simulink model "SF045A_HwAgSysArbn"  (R2013b)
settings: Solver=FixedStepDiscrete  SolverMode=SingleTasking  StartTime=0.0  StopTime=1  FixedStep=.002  RelTol=1e-3
values from neighbouring files (symbols this model uses):
  ARCHGLBPRM_2MILLISEC_SEC_F32 = DataDict.Constant    [SF045A_HwAgSysArbn_DataDict.m]
  CNVSECTOCNT_CNTPERSEC_U32 = DataDict.Constant    [SF045A_HwAgSysArbn_DataDict.m]
  CNVTOMILLISEC_MILLISECPERCNT_F32 = DataDict.Constant    [SF045A_HwAgSysArbn_DataDict.m]
  FltInj_f32 = DataDict.Client    [SF045A_HwAgSysArbn_DataDict.m]
  FLTINJ_HWAGSYSARBN_HWAG = DataDict.Constant    [SF045A_HwAgSysArbn_DataDict.m]
  FLTINJ_HWAGSYSARBN_SERLCOMHWAG = DataDict.Constant    [SF045A_HwAgSysArbn_DataDict.m]
  HwAgSysArbnHwAgConf1Snsr = DataDict.Calibration    [SF045A_HwAgSysArbn_DataDict.m]
  HwAgSysArbnHwAgConf2Snsr = DataDict.Calibration    [SF045A_HwAgSysArbn_DataDict.m]
  HwAgSysArbnHwAgConfNoSnsr = DataDict.Calibration    [SF045A_HwAgSysArbn_DataDict.m]
  HwAgSysArbnHwAgCorrdCorrlnThd = DataDict.Calibration    [SF045A_HwAgSysArbn_DataDict.m]
  HwAgSysArbnHwAgCorrlnFailDebStep = DataDict.Calibration    [SF045A_HwAgSysArbn_DataDict.m]
  HwAgSysArbnHwAgCorrlnPassDebStep = DataDict.Calibration    [SF045A_HwAgSysArbn_DataDict.m]
  HwAgSysArbnHwAgCorrlnRng = DataDict.Calibration    [SF045A_HwAgSysArbn_DataDict.m]
  HwAgSysArbnHwAgSlewRate = DataDict.Calibration    [SF045A_HwAgSysArbn_DataDict.m]
  HwAgSysArbnHwAgSnsrlsCorrlnThd = DataDict.Calibration    [SF045A_HwAgSysArbn_DataDict.m]
  HwAgSysArbnHwAgSnsrlsKineThd = DataDict.Calibration    [SF045A_HwAgSysArbn_DataDict.m]
  HwAgSysArbnHwAgToMotAgCorrlnElpdTiLim = DataDict.Calibration    [SF045A_HwAgSysArbn_DataDict.m]
  HwAgSysArbnSerlComHwAgCorrdConf = DataDict.Calibration    [SF045A_HwAgSysArbn_DataDict.m]
  HwAgSysArbnSerlComHwAgSnsrlsConf = DataDict.Calibration    [SF045A_HwAgSysArbn_DataDict.m]
  HwAgSysArbnSlewRateTmr = DataDict.Calibration    [SF045A_HwAgSysArbn_DataDict.m]
  HWAGTHD_ULS_FLOAT32 = DataDict.Constant    [SF045A_HwAgSysArbn_DataDict.m]
  INVLDSRC_CNT_S08 = DataDict.Constant    [SF045A_HwAgSysArbn_DataDict.m]
  LRGSLEW_HWDEGPERSEC_F32 = DataDict.Constant    [SF045A_HwAgSysArbn_DataDict.m]
  NODEBSTEP_CNT_U16 = DataDict.Constant    [SF045A_HwAgSysArbn_DataDict.m]
  SLEWINPROGS_CNT_LGC = DataDict.Constant    [SF045A_HwAgSysArbn_DataDict.m]
  SLEWNOTINPROGS_CNT_LGC = DataDict.Constant    [SF045A_HwAgSysArbn_DataDict.m]
  SNSRDATASRCSELD_CNT_S08 = DataDict.Constant    [SF045A_HwAgSysArbn_DataDict.m]
  SNSRLSDATASRCSELD_CNT_S08 = DataDict.Constant    [SF045A_HwAgSysArbn_DataDict.m]
  ZEROTMR_MILLISEC_F32 = DataDict.Constant    [SF045A_HwAgSysArbn_DataDict.m]
undefined symbols (not defined in the file or in its folder): NtcNr1, NtcSts1
libraries: simulink x10, NxtrLim x7, autosarlib x2, NxtrAbslt x2
(part 3 of 3)

== system SF045A_HwAgSysArbn/HwAgSysArbn/HwAgSysArbnPer1/HwAgArbn/HwAgSrcSeln/ChkCorrln/SetNtcPass ==
  Action Port : ActionPort  ActionType=then
  Constant15 : Constant  RequirementInfo={} %GIDa_eeb50086_ebb6_4513_9847_6cae94a7ac91  Value=HwAgSysArbnHwAgCorrlnPassDebStep
  Constant18 : Constant  RequirementInfo={} %GIDa_013e9517_c477_4830_bdf4_1b47d908796e  Value=0
  Constant4 : Constant  RequirementInfo={} %GIDa_90515fd1_2125_4550_9fa1_625f6dc30aa8  Value=true  OutDataTypeStr=boolean
      settings: AttributesFormatString=%<OutDataTypeStr>
  CopyRight2 : Subsystem  Description=|  mask(Copyright Information){none=on}
      | Copyright info block.                                               
      |                                                                     
      | Place copyright information at the top of every subsystem in design.
      mask prompts: none "No parameters"
      mask help: Place copyright information at the top of every subsystem in design.
      mask Display:
      | NxtrConf = 'Nexteer Confidential';
      | 
      | sys = bdroot; %handle for the current model ("system")
      | first = get_param(sys,'Created');
      | first = first(end-3:end);  %year is last four digits
      | 
      | last = get_param(sys,'LastModifiedDate');
      | if isempty(last)
      |     last = datestr(now,'yyyy');
      | else
      |     last = last(end-3:end);
      | end
      | 
      | if strcmp(first,last)
      |     fprintf('%s -- Copyright %s Nexteer',NxtrConf,first)
      | else
      |     fprintf('%s -- %s%s- %s Nexteer',NxtrConf,char(169),first,last)
      | end
  Data Store Write1 : DataStoreWrite  RequirementInfo={} %GIDa_5a1ff29e_b92d_44ac_baea_bdad4ffa5dd1  DataStoreName=HwAgToMotAgCorrlnDurnRefTmr
  Data Store Write3 : DataStoreWrite  RequirementInfo={} %GIDa_9a2b2c1d_b743_4844_a03a_8556aaa946e3  DataStoreName=HwAgToMotAgCorrln
  Enumerated Constant13 : simulink/Sources/Enumerated Constant  RequirementInfo={} %GIDa_0b00377d_3f79_4e44_b7d4_456cdb84d0e3  OutDataTypeStr=Enum: NtcSts1  Value=NtcSts1.NTCSTS_PREPASSD  SampleTime=inf
  Enumerated Constant15 : simulink/Sources/Enumerated Constant  RequirementInfo={} %GIDa_b1678220_307d_46cf_99b1_3b05cdcccb07  OutDataTypeStr=Enum: NtcNr1  Value=NtcNr1.NTCNR_0X0A6  SampleTime=inf
  GetRefTmr100MicroSec32bit : Subsystem  RequirementInfo={} %GIDa_050abb2d_d94a_4647_9003_ba1ceee815fb
  SetNtcPass : Subsystem  RequirementInfo={} %GIDa_56eadc5f_fb1c_4ab9_8fbe_9c5bb2cbb9bf  mask(SetNTC){}
      mask help: SetNTC library block
  wires:
  Constant15/1 -> SetNtcPass/4(DebStep)
  Enumerated Constant13/1 -> SetNtcPass/3(NtcSts)
  Constant18/1 -> SetNtcPass/2(NtcStInfo)
  Enumerated Constant15/1 -> SetNtcPass/1(NtcNr)
  Constant4/1 -> Data Store Write3/1
  GetRefTmr100MicroSec32bit/1(RefTmr) -> Data Store Write1/1

== system SF045A_HwAgSysArbn/HwAgSysArbn/HwAgSysArbnPer1/HwAgArbn/HwAgSrcSeln/NoHwAgDataToSerlCom/CopyRight2 ==

== system SF045A_HwAgSysArbn/HwAgSysArbn/HwAgSysArbnPer1/HwAgArbn/HwAgSrcSeln/SnsrDataToSerlCom/CopyRight2 ==

== system SF045A_HwAgSysArbn/HwAgSysArbn/HwAgSysArbnPer1/HwAgArbn/HwAgSrcSeln/SnsrlsDataToSerlCom/CopyRight2 ==

== system SF045A_HwAgSysArbn/HwAgSysArbn/HwAgSysArbnPer1/HwAgArbn/HwAgSrcSeln/SnsrlsDataToSerlCom/CorrlnStsFalse ==
  Action Port : ActionPort  ActionType=else
  Constant1 : Constant  RequirementInfo={} %GIDa_c7135156_251f_40b0_8356_b5a0132d025b  Value=0  OutDataTypeStr=single
      settings: AttributesFormatString=%<OutDataTypeStr>
  Constant3 : Constant  RequirementInfo={} %GIDa_afd38917_26d9_466b_8fc0_bc806b5335e9  Value=0  OutDataTypeStr=boolean
      settings: AttributesFormatString=%<OutDataTypeStr>
  CopyRight2 : Subsystem  Description=|  mask(Copyright Information){none=on}
      | Copyright info block.                                               
      |                                                                     
      | Place copyright information at the top of every subsystem in design.
      mask prompts: none "No parameters"
      mask help: Place copyright information at the top of every subsystem in design.
      mask Display:
      | NxtrConf = 'Nexteer Confidential';
      | 
      | sys = bdroot; %handle for the current model ("system")
      | first = get_param(sys,'Created');
      | first = first(end-3:end);  %year is last four digits
      | 
      | last = get_param(sys,'LastModifiedDate');
      | if isempty(last)
      |     last = datestr(now,'yyyy');
      | else
      |     last = last(end-3:end);
      | end
      | 
      | if strcmp(first,last)
      |     fprintf('%s -- Copyright %s Nexteer',NxtrConf,first)
      | else
      |     fprintf('%s -- %s%s- %s Nexteer',NxtrConf,char(169),first,last)
      | end
  HwAgToSerlCom : Outport  RequirementInfo={} %GIDa_dfac9b99_a6ce_41fa_a1af_5a78eaec718f
  HwAgStsToSerlCom : Outport  RequirementInfo={} %GIDa_a5794653_43a3_4f48_8d32_c475f5222fa0  Port=2
  wires:
  Constant3/1 -> HwAgStsToSerlCom/1
  Constant1/1 -> HwAgToSerlCom/1

== system SF045A_HwAgSysArbn/HwAgSysArbn/HwAgSysArbnPer1/HwAgArbn/HwAgSrcSeln/SnsrlsDataToSerlCom/CorrlnStsTrue ==
  HwAgSnsrls : Inport
  HwAgSnsrlsConf : Inport  Port=2
  Action Port : ActionPort  ActionType=then
  Constant8 : Constant  RequirementInfo={} %GIDa_349ca605_e3c4_4ce4_8a04_8b4b7b6ac69d  Value=HwAgSysArbnSerlComHwAgSnsrlsConf
  CopyRight2 : Subsystem  Description=|  mask(Copyright Information){none=on}
      | Copyright info block.                                               
      |                                                                     
      | Place copyright information at the top of every subsystem in design.
      mask prompts: none "No parameters"
      mask help: Place copyright information at the top of every subsystem in design.
      mask Display:
      | NxtrConf = 'Nexteer Confidential';
      | 
      | sys = bdroot; %handle for the current model ("system")
      | first = get_param(sys,'Created');
      | first = first(end-3:end);  %year is last four digits
      | 
      | last = get_param(sys,'LastModifiedDate');
      | if isempty(last)
      |     last = datestr(now,'yyyy');
      | else
      |     last = last(end-3:end);
      | end
      | 
      | if strcmp(first,last)
      |     fprintf('%s -- Copyright %s Nexteer',NxtrConf,first)
      | else
      |     fprintf('%s -- %s%s- %s Nexteer',NxtrConf,char(169),first,last)
      | end
  Relational Operator : RelationalOperator  RequirementInfo={} %GIDa_03f84a5a_5c25_4fbe_b033_45a585c8ca69  OutDataTypeStr=boolean
  HwAgToSerlCom : Outport
  HwAgStsToSerlCom : Outport  Port=2
  wires:
  Relational Operator/1 -> HwAgStsToSerlCom/1
  Constant8/1 -> Relational Operator/2
  HwAgSnsrlsConf/1 -> Relational Operator/1
  HwAgSnsrls/1 -> HwAgToSerlCom/1

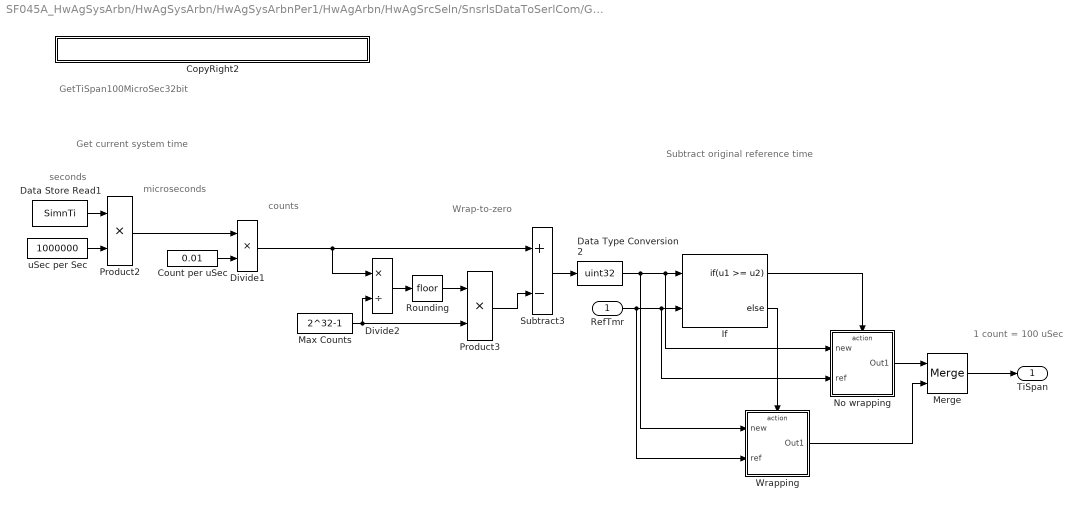
== system SF045A_HwAgSysArbn/HwAgSysArbn/HwAgSysArbnPer1/HwAgArbn/HwAgSrcSeln/SnsrlsDataToSerlCom/GetTiSpan100MicroSec32bit ==
  note: Subtract original reference time
  note: seconds
  note: microseconds
  note: counts
  note: Wrap-to-zero
  note: 1 count = 100 uSec
  note: Get current system time
  note: GetTiSpan100MicroSec32bit
  RefTmr : Inport
  CopyRight2 : Subsystem  Description=|  mask(Copyright Information){none=on}
      | Copyright info block.                                               
      |                                                                     
      | Place copyright information at the top of every subsystem in design.
      mask prompts: none "No parameters"
      mask help: Place copyright information at the top of every subsystem in design.
      mask Display:
      | NxtrConf = 'Nexteer Confidential';
      | 
      | sys = bdroot; %handle for the current model ("system")
      | first = get_param(sys,'Created');
      | if(isempty(first))
      |     first = datestr(now,'yyyy');
      | else
      |     first = first(end-3:end);  %year is last four digits
      | end
      | 
      | last = get_param(sys,'LastModifiedDate');
      | if isempty(last)
      |     last = datestr(now,'yyyy');
      | else
      |     last = last(end-3:end);
      | end
      | 
      | if strcmp(first,last)
      |     fprintf('%s -- Copyright %s Nexteer',NxtrConf,first)
      | else
      |     fprintf('%s -- %s%s- %s Nexteer',NxtrConf,char(169),first,last)
      | end
  Count per uSec : Constant  Value=0.01
  Data Store Read1 : DataStoreRead  DataStoreName=SimnTi
  Data Type Conversion2 : DataTypeConversion  OutDataTypeStr=uint32
  Divide1 : Product  Inputs=**
  Divide2 : Product  Inputs=*/
  If : If  NumInputs=2  IfExpression=u1 >= u2
  Max Counts : Constant  Value=2^32-1
  Merge : Merge
  No wrapping : Subsystem  TreatAsAtomicUnit=on
  Product2 : Product
  Product3 : Product
  Rounding : Rounding
  Subtract3 : Sum  Inputs=+-
  Wrapping : Subsystem  TreatAsAtomicUnit=on
  uSec per Sec : Constant  Value=1000000
  TiSpan : Outport
  wires:
  Wrapping/1(Out1) -> Merge/2
  No wrapping/1(Out1) -> Merge/1
  If/2 -> Wrapping/Action
  If/1 -> No wrapping/Action
  Product3/1 -> Subtract3/2
  Subtract3/1 -> Data Type Conversion2/1
  Rounding/1 -> Product3/1
  Divide2/1 -> Rounding/1
  Max Counts/1 -> Divide2/2, Product3/2
  Divide1/1 -> Divide2/1, Subtract3/1
  Product2/1 -> Divide1/1
  Data Store Read1/1 -> Product2/1
  Count per uSec/1 -> Divide1/2
  uSec per Sec/1 -> Product2/2
  Merge/1 -> TiSpan/1
  RefTmr/1 -> If/2, No wrapping/2(ref), Wrapping/2(ref)
  Data Type Conversion2/1 -> If/1, No wrapping/1(new), Wrapping/1(new)

== system SF045A_HwAgSysArbn/HwAgSysArbn/HwAgSysArbnPer1/HwAgArbn/HwAgSrcSeln/SnsrlsHwAgSeln/CopyRight2 ==

== system SF045A_HwAgSysArbn/HwAgSysArbn/HwAgSysArbnPer1/HwAgArbn/HwAgSrcSeln/VrfyHwAgCorrln/CopyRight2 ==

== system SF045A_HwAgSysArbn/HwAgSysArbn/HwAgSysArbnPer1/HwAgArbn/TestHwAgSrcChg/ RetainSlewRate/CopyRight2 ==

== system SF045A_HwAgSysArbn/HwAgSysArbn/HwAgSysArbnPer1/HwAgArbn/TestHwAgSrcChg/ApplyLrgSlew/CopyRight2 ==

== system SF045A_HwAgSysArbn/HwAgSysArbn/HwAgSysArbnPer1/HwAgArbn/TestHwAgSrcChg/ApplyRateLim/ RetainHwAgConf ==
  note: Pass on the previous values of Hw Ag Confidence as Slewing is not complete
  PrevHwAgConf : Inport
  Action Port : ActionPort  ActionType=then
  Constant4 : Constant  Value=SLEWINPROGS_CNT_LGC
  CopyRight2 : Subsystem  Description=|  mask(Copyright Information){none=on}
      | Copyright info block.                                               
      |                                                                     
      | Place copyright information at the top of every subsystem in design.
      mask prompts: none "No parameters"
      mask help: Place copyright information at the top of every subsystem in design.
      mask Display:
      | NxtrConf = 'Nexteer Confidential';
      | 
      | sys = bdroot; %handle for the current model ("system")
      | first = get_param(sys,'Created');
      | first = first(end-3:end);  %year is last four digits
      | 
      | last = get_param(sys,'LastModifiedDate');
      | if isempty(last)
      |     last = datestr(now,'yyyy');
      | else
      |     last = last(end-3:end);
      | end
      | 
      | if strcmp(first,last)
      |     fprintf('%s -- Copyright %s Nexteer',NxtrConf,first)
      | else
      |     fprintf('%s -- %s%s- %s Nexteer',NxtrConf,char(169),first,last)
      | end
  Data Store Write5 : DataStoreWrite  RequirementInfo={} %GIDa_e610268f_4251_4a50_930a_b136411808b8  DataStoreName=SlewSts
  "HwAgConf " : Outport
  wires:
  PrevHwAgConf/1 -> "HwAgConf "/1
  Constant4/1 -> Data Store Write5/1

== system SF045A_HwAgSysArbn/HwAgSysArbn/HwAgSysArbnPer1/HwAgArbn/TestHwAgSrcChg/ApplyRateLim/CopyRight2 ==

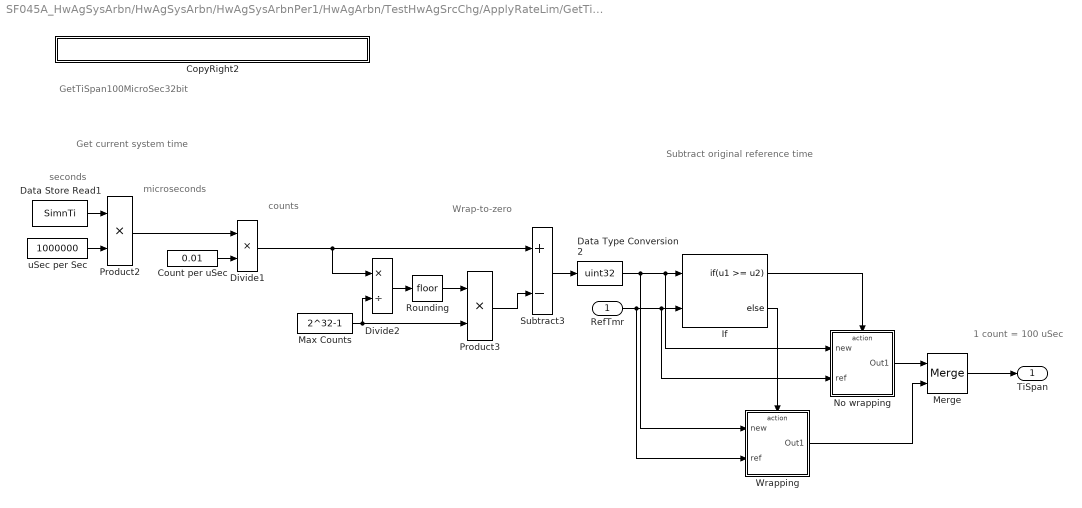
== system SF045A_HwAgSysArbn/HwAgSysArbn/HwAgSysArbnPer1/HwAgArbn/TestHwAgSrcChg/ApplyRateLim/GetTiSpan100MicroSec32bit ==
  note: Subtract original reference time
  note: seconds
  note: microseconds
  note: counts
  note: Wrap-to-zero
  note: 1 count = 100 uSec
  note: Get current system time
  note: GetTiSpan100MicroSec32bit
  RefTmr : Inport
  CopyRight2 : Subsystem  Description=|  mask(Copyright Information){none=on}
      | Copyright info block.                                               
      |                                                                     
      | Place copyright information at the top of every subsystem in design.
      mask prompts: none "No parameters"
      mask help: Place copyright information at the top of every subsystem in design.
      mask Display:
      | NxtrConf = 'Nexteer Confidential';
      | 
      | sys = bdroot; %handle for the current model ("system")
      | first = get_param(sys,'Created');
      | if(isempty(first))
      |     first = datestr(now,'yyyy');
      | else
      |     first = first(end-3:end);  %year is last four digits
      | end
      | 
      | last = get_param(sys,'LastModifiedDate');
      | if isempty(last)
      |     last = datestr(now,'yyyy');
      | else
      |     last = last(end-3:end);
      | end
      | 
      | if strcmp(first,last)
      |     fprintf('%s -- Copyright %s Nexteer',NxtrConf,first)
      | else
      |     fprintf('%s -- %s%s- %s Nexteer',NxtrConf,char(169),first,last)
      | end
  Count per uSec : Constant  Value=0.01
  Data Store Read1 : DataStoreRead  DataStoreName=SimnTi
  Data Type Conversion2 : DataTypeConversion  OutDataTypeStr=uint32
  Divide1 : Product  Inputs=**
  Divide2 : Product  Inputs=*/
  If : If  NumInputs=2  IfExpression=u1 >= u2
  Max Counts : Constant  Value=2^32-1
  Merge : Merge
  No wrapping : Subsystem  TreatAsAtomicUnit=on
  Product2 : Product
  Product3 : Product
  Rounding : Rounding
  Subtract3 : Sum  Inputs=+-
  Wrapping : Subsystem  TreatAsAtomicUnit=on
  uSec per Sec : Constant  Value=1000000
  TiSpan : Outport
  wires:
  Wrapping/1(Out1) -> Merge/2
  No wrapping/1(Out1) -> Merge/1
  If/2 -> Wrapping/Action
  If/1 -> No wrapping/Action
  Product3/1 -> Subtract3/2
  Subtract3/1 -> Data Type Conversion2/1
  Rounding/1 -> Product3/1
  Divide2/1 -> Rounding/1
  Max Counts/1 -> Divide2/2, Product3/2
  Divide1/1 -> Divide2/1, Subtract3/1
  Product2/1 -> Divide1/1
  Data Store Read1/1 -> Product2/1
  Count per uSec/1 -> Divide1/2
  uSec per Sec/1 -> Product2/2
  Merge/1 -> TiSpan/1
  RefTmr/1 -> If/2, No wrapping/2(ref), Wrapping/2(ref)
  Data Type Conversion2/1 -> If/1, No wrapping/1(new), Wrapping/1(new)

== system SF045A_HwAgSysArbn/HwAgSysArbn/HwAgSysArbnPer1/HwAgArbn/TestHwAgSrcChg/ApplyRateLim/Pass ==
  note: Pass on the computed values of Hw Ag Confidence as Slewing is not in progress
  HwAgConfInp : Inport
  Action Port : ActionPort  ActionType=else
  Constant4 : Constant  Value=SLEWNOTINPROGS_CNT_LGC
  CopyRight2 : Subsystem  Description=|  mask(Copyright Information){none=on}
      | Copyright info block.                                               
      |                                                                     
      | Place copyright information at the top of every subsystem in design.
      mask prompts: none "No parameters"
      mask help: Place copyright information at the top of every subsystem in design.
      mask Display:
      | NxtrConf = 'Nexteer Confidential';
      | 
      | sys = bdroot; %handle for the current model ("system")
      | first = get_param(sys,'Created');
      | first = first(end-3:end);  %year is last four digits
      | 
      | last = get_param(sys,'LastModifiedDate');
      | if isempty(last)
      |     last = datestr(now,'yyyy');
      | else
      |     last = last(end-3:end);
      | end
      | 
      | if strcmp(first,last)
      |     fprintf('%s -- Copyright %s Nexteer',NxtrConf,first)
      | else
      |     fprintf('%s -- %s%s- %s Nexteer',NxtrConf,char(169),first,last)
      | end
  Data Store Write5 : DataStoreWrite  RequirementInfo={} %GIDa_e00d6d32_3e14_4362_9726_dd90d4df3b91  DataStoreName=SlewSts
  "HwAgConf " : Outport
  wires:
  HwAgConfInp/1 -> "HwAgConf "/1
  Constant4/1 -> Data Store Write5/1

== system SF045A_HwAgSysArbn/HwAgSysArbn/HwAgSysArbnPer1/HwAgArbn/TestHwAgSrcChg/SetSlewRate/CopyRight2 ==

== system SF045A_HwAgSysArbn/HwAgSysArbn/HwAgSysArbnPer1/HwAgArbn/TestHwAgSrcChg/SetSlewRate/GetRefTmr100MicroSec32bit ==
  note: 1 count = 100 uSec
  note: seconds
  note: microseconds
  note: counts
  note: Wrap-to-zero
  note: GetRefTmr100MicroSec32bit
  CopyRight2 : Subsystem  Description=|  mask(Copyright Information){none=on}
      | Copyright info block.                                               
      |                                                                     
      | Place copyright information at the top of every subsystem in design.
      mask prompts: none "No parameters"
      mask help: Place copyright information at the top of every subsystem in design.
      mask Display:
      | NxtrConf = 'Nexteer Confidential';
      | 
      | sys = bdroot; %handle for the current model ("system")
      | first = get_param(sys,'Created');
      | if(isempty(first))
      |     first = datestr(now,'yyyy');
      | else
      |     first = first(end-3:end);  %year is last four digits
      | end
      | 
      | last = get_param(sys,'LastModifiedDate');
      | if isempty(last)
      |     last = datestr(now,'yyyy');
      | else
      |     last = last(end-3:end);
      | end
      | 
      | if strcmp(first,last)
      |     fprintf('%s -- Copyright %s Nexteer',NxtrConf,first)
      | else
      |     fprintf('%s -- %s%s- %s Nexteer',NxtrConf,char(169),first,last)
      | end
  Count per uSec : Constant  Value=0.01
  Data Store Read1 : DataStoreRead  DataStoreName=SimnTi
  Data Type Conversion1 : DataTypeConversion  OutDataTypeStr=uint32
  Divide1 : Product  Inputs=**
  Divide2 : Product  Inputs=*/
  Max Counts : Constant  Value=2^32-1
  Product1 : Product
  Product2 : Product
  Rounding : Rounding
  Subtract1 : Sum  Inputs=+-
  uSec per Sec : Constant  Value=1000000
  RefTmr : Outport
  wires:
  Product2/1 -> Subtract1/2
  Subtract1/1 -> Data Type Conversion1/1
  Rounding/1 -> Product2/1
  Divide2/1 -> Rounding/1
  Max Counts/1 -> Divide2/2, Product2/2
  Divide1/1 -> Divide2/1, Subtract1/1
  Product1/1 -> Divide1/1
  Data Store Read1/1 -> Product1/1
  Count per uSec/1 -> Divide1/2
  uSec per Sec/1 -> Product1/2
  Data Type Conversion1/1 -> RefTmr/1

== system SF045A_HwAgSysArbn/HwAgSysArbn/HwAgSysArbnPer1/HwAgArbn/VldtSnsrlsData/Pass/CopyRight2 ==

== system SF045A_HwAgSysArbn/HwAgSysArbn/HwAgSysArbnPer1/HwAgArbn/VldtSnsrlsData/ThdExcdd/CopyRight2 ==

== system SF045A_HwAgSysArbn/HwAgSysArbn/HwAgSysArbnPer1/HwAgArbn/VldtSnsrlsData/ThdExcdd/Kinematic Integrity ==
  NtcNr : Inport
  NtcStInfo : Inport  Port=2
  NtcSts : Inport  Port=3
  DebStep : Inport  Port=4
  SetNtcSts : Subsystem  RequirementInfo={} %GIDa_58144789_61c4_4a7b_8c14_60385a32cfb3  TreatAsAtomicUnit=on
      settings: RTWSystemCode=Inline
  wires:
  NtcStInfo/1 -> SetNtcSts/2(NtcStInfo)
  DebStep/1 -> SetNtcSts/4(DebStep)
  NtcSts/1 -> SetNtcSts/3(NtcSts)
  NtcNr/1 -> SetNtcSts/1(NtcNr)  "NtcNr"

== system SF045A_HwAgSysArbn/HwAgSysArbn/HwAgSysArbnPer1/HwAgArbn/HwAgSrcSeln/ChkCorrln/SetCorrlFltNtc/CopyRight2 ==

== system SF045A_HwAgSysArbn/HwAgSysArbn/HwAgSysArbnPer1/HwAgArbn/HwAgSrcSeln/ChkCorrln/SetCorrlFltNtc/SetCorrlFltNtc ==
  NtcNr : Inport
  NtcStInfo : Inport  Port=2
  NtcSts : Inport  Port=3
  DebStep : Inport  Port=4
  SetNtcSts : Subsystem  RequirementInfo={} %GIDa_0a5e138f_bbbe_4d9e_8ebe_c8090c91025c  TreatAsAtomicUnit=on
      settings: RTWSystemCode=Inline
  wires:
  NtcStInfo/1 -> SetNtcSts/2(NtcStInfo)
  DebStep/1 -> SetNtcSts/4(DebStep)
  NtcSts/1 -> SetNtcSts/3(NtcSts)
  NtcNr/1 -> SetNtcSts/1(NtcNr)  "NtcNr"

== system SF045A_HwAgSysArbn/HwAgSysArbn/HwAgSysArbnPer1/HwAgArbn/HwAgSrcSeln/ChkCorrln/SetNtcPass/CopyRight2 ==

== system SF045A_HwAgSysArbn/HwAgSysArbn/HwAgSysArbnPer1/HwAgArbn/HwAgSrcSeln/ChkCorrln/SetNtcPass/GetRefTmr100MicroSec32bit ==
  note: 1 count = 100 uSec
  note: seconds
  note: microseconds
  note: counts
  note: Wrap-to-zero
  note: GetRefTmr100MicroSec32bit
  CopyRight2 : Subsystem  Description=|  mask(Copyright Information){none=on}
      | Copyright info block.                                               
      |                                                                     
      | Place copyright information at the top of every subsystem in design.
      mask prompts: none "No parameters"
      mask help: Place copyright information at the top of every subsystem in design.
      mask Display:
      | NxtrConf = 'Nexteer Confidential';
      | 
      | sys = bdroot; %handle for the current model ("system")
      | first = get_param(sys,'Created');
      | if(isempty(first))
      |     first = datestr(now,'yyyy');
      | else
      |     first = first(end-3:end);  %year is last four digits
      | end
      | 
      | last = get_param(sys,'LastModifiedDate');
      | if isempty(last)
      |     last = datestr(now,'yyyy');
      | else
      |     last = last(end-3:end);
      | end
      | 
      | if strcmp(first,last)
      |     fprintf('%s -- Copyright %s Nexteer',NxtrConf,first)
      | else
      |     fprintf('%s -- %s%s- %s Nexteer',NxtrConf,char(169),first,last)
      | end
  Count per uSec : Constant  Value=0.01
  Data Store Read1 : DataStoreRead  DataStoreName=SimnTi
  Data Type Conversion1 : DataTypeConversion  OutDataTypeStr=uint32
  Divide1 : Product  Inputs=**
  Divide2 : Product  Inputs=*/
  Max Counts : Constant  Value=2^32-1
  Product1 : Product
  Product2 : Product
  Rounding : Rounding
  Subtract1 : Sum  Inputs=+-
  uSec per Sec : Constant  Value=1000000
  RefTmr : Outport
  wires:
  Product2/1 -> Subtract1/2
  Subtract1/1 -> Data Type Conversion1/1
  Rounding/1 -> Product2/1
  Divide2/1 -> Rounding/1
  Max Counts/1 -> Divide2/2, Product2/2
  Divide1/1 -> Divide2/1, Subtract1/1
  Product1/1 -> Divide1/1
  Data Store Read1/1 -> Product1/1
  Count per uSec/1 -> Divide1/2
  uSec per Sec/1 -> Product1/2
  Data Type Conversion1/1 -> RefTmr/1

== system SF045A_HwAgSysArbn/HwAgSysArbn/HwAgSysArbnPer1/HwAgArbn/HwAgSrcSeln/ChkCorrln/SetNtcPass/SetNtcPass ==
  NtcNr : Inport
  NtcStInfo : Inport  Port=2
  NtcSts : Inport  Port=3
  DebStep : Inport  Port=4
  SetNtcSts : Subsystem  RequirementInfo={} %GIDa_17711836_ebc0_49f1_9698_b758e03a4efd  TreatAsAtomicUnit=on
      settings: RTWSystemCode=Inline
  wires:
  NtcNr/1 -> SetNtcSts/1(NtcNr)  "NtcNr"
  NtcSts/1 -> SetNtcSts/3(NtcSts)
  DebStep/1 -> SetNtcSts/4(DebStep)
  NtcStInfo/1 -> SetNtcSts/2(NtcStInfo)

== system SF045A_HwAgSysArbn/HwAgSysArbn/HwAgSysArbnPer1/HwAgArbn/HwAgSrcSeln/SnsrlsDataToSerlCom/CorrlnStsFalse/CopyRight2 ==

== system SF045A_HwAgSysArbn/HwAgSysArbn/HwAgSysArbnPer1/HwAgArbn/HwAgSrcSeln/SnsrlsDataToSerlCom/CorrlnStsTrue/CopyRight2 ==

== system SF045A_HwAgSysArbn/HwAgSysArbn/HwAgSysArbnPer1/HwAgArbn/HwAgSrcSeln/SnsrlsDataToSerlCom/GetTiSpan100MicroSec32bit/CopyRight2 ==

== system SF045A_HwAgSysArbn/HwAgSysArbn/HwAgSysArbnPer1/HwAgArbn/HwAgSrcSeln/SnsrlsDataToSerlCom/GetTiSpan100MicroSec32bit/No wrapping ==
  new : Inport
  ref : Inport  Port=2
  Action Port : ActionPort  ActionType=then
  Subtract1 : Sum  Inputs=+-
  Out1 : Outport
  wires:
  ref/1 -> Subtract1/2
  new/1 -> Subtract1/1
  Subtract1/1 -> Out1/1

== system SF045A_HwAgSysArbn/HwAgSysArbn/HwAgSysArbnPer1/HwAgArbn/HwAgSrcSeln/SnsrlsDataToSerlCom/GetTiSpan100MicroSec32bit/Wrapping ==
  new : Inport
  ref : Inport  Port=2
  Action Port : ActionPort  ActionType=else
  Max Counts : Constant  Value=2^32-1  OutDataTypeStr=uint32
  Subtract1 : Sum  Inputs=+-+
  Out1 : Outport
  wires:
  new/1 -> Subtract1/3
  ref/1 -> Subtract1/2
  Max Counts/1 -> Subtract1/1
  Subtract1/1 -> Out1/1

== system SF045A_HwAgSysArbn/HwAgSysArbn/HwAgSysArbnPer1/HwAgArbn/TestHwAgSrcChg/ApplyRateLim/ RetainHwAgConf/CopyRight2 ==

== system SF045A_HwAgSysArbn/HwAgSysArbn/HwAgSysArbnPer1/HwAgArbn/TestHwAgSrcChg/ApplyRateLim/GetTiSpan100MicroSec32bit/CopyRight2 ==

== system SF045A_HwAgSysArbn/HwAgSysArbn/HwAgSysArbnPer1/HwAgArbn/TestHwAgSrcChg/ApplyRateLim/GetTiSpan100MicroSec32bit/No wrapping ==
  new : Inport
  ref : Inport  Port=2
  Action Port : ActionPort  ActionType=then
  Subtract1 : Sum  Inputs=+-
  Out1 : Outport
  wires:
  ref/1 -> Subtract1/2
  new/1 -> Subtract1/1
  Subtract1/1 -> Out1/1

== system SF045A_HwAgSysArbn/HwAgSysArbn/HwAgSysArbnPer1/HwAgArbn/TestHwAgSrcChg/ApplyRateLim/GetTiSpan100MicroSec32bit/Wrapping ==
  new : Inport
  ref : Inport  Port=2
  Action Port : ActionPort  ActionType=else
  Max Counts : Constant  Value=2^32-1  OutDataTypeStr=uint32
  Subtract1 : Sum  Inputs=+-+
  Out1 : Outport
  wires:
  new/1 -> Subtract1/3
  ref/1 -> Subtract1/2
  Max Counts/1 -> Subtract1/1
  Subtract1/1 -> Out1/1

== system SF045A_HwAgSysArbn/HwAgSysArbn/HwAgSysArbnPer1/HwAgArbn/TestHwAgSrcChg/ApplyRateLim/Pass/CopyRight2 ==

== system SF045A_HwAgSysArbn/HwAgSysArbn/HwAgSysArbnPer1/HwAgArbn/TestHwAgSrcChg/SetSlewRate/GetRefTmr100MicroSec32bit/CopyRight2 ==

== system SF045A_HwAgSysArbn/HwAgSysArbn/HwAgSysArbnPer1/HwAgArbn/VldtSnsrlsData/ThdExcdd/Kinematic Integrity/SetNtcSts ==
  note: Note:
      |
      | - "ISO Fault Debounce Design" Simulink block intent to use here for Simulation purpose only. Do not Code this block
  NtcNr : Inport
  NtcStInfo : Inport  Port=2
  NtcSts : Inport  Port=3
  DebStep : Inport  Port=4
  CopyRight2 : Subsystem  Description=|  mask(Copyright Information){none=on}
      | Copyright info block.                                               
      |                                                                     
      | Place copyright information at the top of every subsystem in design.
      mask prompts: none "No parameters"
      mask help: Place copyright information at the top of every subsystem in design.
      mask Display:
      | NxtrConf = 'Nexteer Confidential';
      | 
      | sys = bdroot; %handle for the current model ("system")
      | first = get_param(sys,'Created');
      | if(isempty(first))
      |     first = datestr(now,'yyyy');
      | else
      |     first = first(end-3:end);  %year is last four digits
      | end
      | 
      | last = get_param(sys,'LastModifiedDate');
      | if isempty(last)
      |     last = datestr(now,'yyyy');
      | else
      |     last = last(end-3:end);
      | end
      | 
      | if strcmp(first,last)
      |     fprintf('%s -- Copyright %s Nexteer',NxtrConf,first)
      | else
      |     fprintf('%s -- %s%s- %s Nexteer',NxtrConf,char(169),first,last)
      | end
  Data Store Write : DataStoreWrite  DataStoreName=NtcQlfr
  Data Store Write1 : DataStoreWrite  DataStoreName=NtcQlfrHwAgSnsrlsThdExcd
  Data Store Write2 : DataStoreWrite  DataStoreName=NtcStInfoHwAgSnsrlsThdExcd
  Data Store Write3 : DataStoreWrite  DataStoreName=NtcStsHwAgSnsrlsThdExcd
  Data Type Conversion : DataTypeConversion  OutDataTypeStr=Enum: SigQlfr1
  Data Type Conversion1 : DataTypeConversion  OutDataTypeStr=uint8
  Ground : Ground
  ISO Fault Debounce Design : Stateflow chart  TreatAsAtomicUnit=on
      settings: AttributesFormatString=|
      | Simulation Purpose Only.
      | Do Not Code this block
      | Diagnostic Manager Owns this requirement
  Terminator : Terminator
  Terminator1 : Terminator
  wires:
  Data Type Conversion1/1 -> Data Store Write2/1
  NtcStInfo/1 -> Terminator1/1, Data Type Conversion1/1
  NtcSts/1 -> ISO Fault Debounce Design/1(NtcSts), Data Store Write3/1
  Data Type Conversion/1 -> Data Store Write/1, Data Store Write1/1
  Ground/1 -> ISO Fault Debounce Design/3(SvcClr)
  ISO Fault Debounce Design/1(Qualifier) -> Data Type Conversion/1
  DebStep/1 -> ISO Fault Debounce Design/2(DebStep)
  NtcNr/1 -> Terminator/1

== system SF045A_HwAgSysArbn/HwAgSysArbn/HwAgSysArbnPer1/HwAgArbn/HwAgSrcSeln/ChkCorrln/SetCorrlFltNtc/SetCorrlFltNtc/SetNtcSts ==
  note: Note:
      |
      | - "ISO Fault Debounce Design" Simulink block intent to use here for Simulation purpose only. Do not Code this block
  NtcNr : Inport
  NtcStInfo : Inport  Port=2
  NtcSts : Inport  Port=3
  DebStep : Inport  Port=4
  CopyRight2 : Subsystem  Description=|  mask(Copyright Information){none=on}
      | Copyright info block.                                               
      |                                                                     
      | Place copyright information at the top of every subsystem in design.
      mask prompts: none "No parameters"
      mask help: Place copyright information at the top of every subsystem in design.
      mask Display:
      | NxtrConf = 'Nexteer Confidential';
      | 
      | sys = bdroot; %handle for the current model ("system")
      | first = get_param(sys,'Created');
      | if(isempty(first))
      |     first = datestr(now,'yyyy');
      | else
      |     first = first(end-3:end);  %year is last four digits
      | end
      | 
      | last = get_param(sys,'LastModifiedDate');
      | if isempty(last)
      |     last = datestr(now,'yyyy');
      | else
      |     last = last(end-3:end);
      | end
      | 
      | if strcmp(first,last)
      |     fprintf('%s -- Copyright %s Nexteer',NxtrConf,first)
      | else
      |     fprintf('%s -- %s%s- %s Nexteer',NxtrConf,char(169),first,last)
      | end
  Data Store Write : DataStoreWrite  DataStoreName=NtcQlfr
  Data Store Write1 : DataStoreWrite  DataStoreName=NtcQlfrHwAgToMotAgCorrln
  Data Store Write2 : DataStoreWrite  DataStoreName=NtcStInfoHwAgToMotAgCorrln
  Data Store Write3 : DataStoreWrite  DataStoreName=NtcStsHwAgToMotAgCorrln
  Data Type Conversion : DataTypeConversion  OutDataTypeStr=Enum: SigQlfr1
  Data Type Conversion1 : DataTypeConversion  OutDataTypeStr=uint8
  Ground : Ground
  ISO Fault Debounce Design : Stateflow chart  TreatAsAtomicUnit=on
      settings: AttributesFormatString=|
      | Simulation Purpose Only.
      | Do Not Code this block
      | Diagnostic Manager Owns this requirement
  Terminator : Terminator
  Terminator1 : Terminator
  wires:
  Data Type Conversion1/1 -> Data Store Write2/1
  NtcStInfo/1 -> Terminator1/1, Data Type Conversion1/1
  NtcSts/1 -> ISO Fault Debounce Design/1(NtcSts), Data Store Write3/1
  Data Type Conversion/1 -> Data Store Write/1, Data Store Write1/1
  Ground/1 -> ISO Fault Debounce Design/3(SvcClr)
  ISO Fault Debounce Design/1(Qualifier) -> Data Type Conversion/1
  DebStep/1 -> ISO Fault Debounce Design/2(DebStep)
  NtcNr/1 -> Terminator/1

== system SF045A_HwAgSysArbn/HwAgSysArbn/HwAgSysArbnPer1/HwAgArbn/HwAgSrcSeln/ChkCorrln/SetNtcPass/GetRefTmr100MicroSec32bit/CopyRight2 ==

== system SF045A_HwAgSysArbn/HwAgSysArbn/HwAgSysArbnPer1/HwAgArbn/HwAgSrcSeln/ChkCorrln/SetNtcPass/SetNtcPass/SetNtcSts ==
  note: Note:
      |
      | - "ISO Fault Debounce Design" Simulink block intent to use here for Simulation purpose only. Do not Code this block
  NtcNr : Inport
  NtcStInfo : Inport  Port=2
  NtcSts : Inport  Port=3
  DebStep : Inport  Port=4
  CopyRight2 : Subsystem  Description=|  mask(Copyright Information){none=on}
      | Copyright info block.                                               
      |                                                                     
      | Place copyright information at the top of every subsystem in design.
      mask prompts: none "No parameters"
      mask help: Place copyright information at the top of every subsystem in design.
      mask Display:
      | NxtrConf = 'Nexteer Confidential';
      | 
      | sys = bdroot; %handle for the current model ("system")
      | first = get_param(sys,'Created');
      | if(isempty(first))
      |     first = datestr(now,'yyyy');
      | else
      |     first = first(end-3:end);  %year is last four digits
      | end
      | 
      | last = get_param(sys,'LastModifiedDate');
      | if isempty(last)
      |     last = datestr(now,'yyyy');
      | else
      |     last = last(end-3:end);
      | end
      | 
      | if strcmp(first,last)
      |     fprintf('%s -- Copyright %s Nexteer',NxtrConf,first)
      | else
      |     fprintf('%s -- %s%s- %s Nexteer',NxtrConf,char(169),first,last)
      | end
  Data Store Write : DataStoreWrite  DataStoreName=NtcQlfr
  Data Store Write1 : DataStoreWrite  DataStoreName=NtcQlfrHwAgToMotAgCorrln
  Data Store Write2 : DataStoreWrite  DataStoreName=NtcStInfoHwAgToMotAgCorrln
  Data Store Write3 : DataStoreWrite  DataStoreName=NtcStsHwAgToMotAgCorrln
  Data Type Conversion : DataTypeConversion  OutDataTypeStr=Enum: SigQlfr1
  Data Type Conversion1 : DataTypeConversion  OutDataTypeStr=uint8
  Ground : Ground
  ISO Fault Debounce Design : Stateflow chart  TreatAsAtomicUnit=on
      settings: AttributesFormatString=|
      | Simulation Purpose Only.
      | Do Not Code this block
      | Diagnostic Manager Owns this requirement
  Terminator : Terminator
  Terminator1 : Terminator
  wires:
  NtcNr/1 -> Terminator/1
  DebStep/1 -> ISO Fault Debounce Design/2(DebStep)
  ISO Fault Debounce Design/1(Qualifier) -> Data Type Conversion/1
  Ground/1 -> ISO Fault Debounce Design/3(SvcClr)
  Data Type Conversion/1 -> Data Store Write1/1, Data Store Write/1
  NtcSts/1 -> Data Store Write3/1, ISO Fault Debounce Design/1(NtcSts)
  NtcStInfo/1 -> Data Type Conversion1/1, Terminator1/1
  Data Type Conversion1/1 -> Data Store Write2/1

== system SF045A_HwAgSysArbn/HwAgSysArbn/HwAgSysArbnPer1/HwAgArbn/VldtSnsrlsData/ThdExcdd/Kinematic Integrity/SetNtcSts/CopyRight2 ==

== system SF045A_HwAgSysArbn/HwAgSysArbn/HwAgSysArbnPer1/HwAgArbn/HwAgSrcSeln/ChkCorrln/SetCorrlFltNtc/SetCorrlFltNtc/SetNtcSts/CopyRight2 ==

== system SF045A_HwAgSysArbn/HwAgSysArbn/HwAgSysArbnPer1/HwAgArbn/HwAgSrcSeln/ChkCorrln/SetNtcPass/SetNtcPass/SetNtcSts/CopyRight2 ==

== stateflow chart SF045A_HwAgSysArbn/HwAgSysArbn/HwAgSysArbnPer1/HwAgArbn/HwAgSrcSeln/ChkCorrln/SetNtcPass/SetNtcPass/SetNtcSts/ISO Fault Debounce Design ==
  note: NTCSTS_PASSD           (0)
      | NTCSTS_FAILD             (1)
      | NTCSTS_PREPASSD   (2)
      | NTCSTS_PREFAILD     (3)
      |
      | SIGQLFR_NORES        (0)
      | SIGQLFR_PASSD         (1)
      | SIGQLFR_FAILD           (2)
  note: Pass Loop
  note: Fail Loop
  note: 
  (default) -> (junction 89)
  (junction 89) -> (junction 95) [order 1] : [NtcSts ==3]
  (junction 89) -> (junction 93) [order 2] : [NtcSts ==2]
  (junction 89) -> (junction 141) [order 3] : [NtcSts ==1]
      | { ErrAcc = 32767;
      | Qualifier =2;
      |  }
  (junction 89) -> (junction 141) [order 4] : [NtcSts ==0]
      | { ErrAcc = -32768;
      | Qualifier=1;
      | }
  (junction 95) -> (junction 103) [order 2]
  (junction 95) -> (junction 111) [order 1] : [ErrAcc <=0]
      | {ErrAcc = DebStep;}
  (junction 93) -> (junction 123) [order 2] : {
      | ErrAcc = ErrAcc - DebStep;
      | }
  (junction 93) -> (junction 123) [order 1] : [(ErrAcc - DebStep) <= -32768]
      | { ErrAcc = -32768;
      | Qualifier=1;
      | }
  (junction 103) -> (junction 111) [order 1] : [(ErrAcc + DebStep) <32767]
      | {ErrAcc = ErrAcc + DebStep;}
  (junction 103) -> (junction 111) [order 2] : {ErrAcc = 32767;
      | Qualifier =2;}
  (junction 123) -> (junction 141)
  (junction 111) -> (junction 141)
  (junction 141) -> (junction 159) [order 2] : {ErrAcc = 0;
      | Qualifier =0;
      | }
  (junction 141) -> (junction 159) [order 1] : [SvcClr ==0]
  data: NtcSts input Enum: NtcSts1; Qualifier output uint8; DebStep input uint16; ErrAcc local single; SvcClr input

== stateflow chart SF045A_HwAgSysArbn/HwAgSysArbn/HwAgSysArbnPer1/HwAgArbn/HwAgSrcSeln/ChkCorrln/SetCorrlFltNtc/SetCorrlFltNtc/SetNtcSts/ISO Fault Debounce Design ==
  note: NTCSTS_PASSD           (0)
      | NTCSTS_FAILD             (1)
      | NTCSTS_PREPASSD   (2)
      | NTCSTS_PREFAILD     (3)
      |
      | SIGQLFR_NORES        (0)
      | SIGQLFR_PASSD         (1)
      | SIGQLFR_FAILD           (2)
  note: Pass Loop
  note: Fail Loop
  note: 
  (default) -> (junction 89)
  (junction 89) -> (junction 95) [order 1] : [NtcSts ==3]
  (junction 89) -> (junction 93) [order 2] : [NtcSts ==2]
  (junction 89) -> (junction 141) [order 3] : [NtcSts ==1]
      | { ErrAcc = 32767;
      | Qualifier =2;
      |  }
  (junction 89) -> (junction 141) [order 4] : [NtcSts ==0]
      | { ErrAcc = -32768;
      | Qualifier=1;
      | }
  (junction 95) -> (junction 103) [order 2]
  (junction 95) -> (junction 111) [order 1] : [ErrAcc <=0]
      | {ErrAcc = DebStep;}
  (junction 93) -> (junction 123) [order 2] : {
      | ErrAcc = ErrAcc - DebStep;
      | }
  (junction 93) -> (junction 123) [order 1] : [(ErrAcc - DebStep) <= -32768]
      | { ErrAcc = -32768;
      | Qualifier=1;
      | }
  (junction 103) -> (junction 111) [order 1] : [(ErrAcc + DebStep) <32767]
      | {ErrAcc = ErrAcc + DebStep;}
  (junction 103) -> (junction 111) [order 2] : {ErrAcc = 32767;
      | Qualifier =2;}
  (junction 123) -> (junction 141)
  (junction 111) -> (junction 141)
  (junction 141) -> (junction 159) [order 2] : {ErrAcc = 0;
      | Qualifier =0;
      | }
  (junction 141) -> (junction 159) [order 1] : [SvcClr ==0]
  data: NtcSts input Enum: NtcSts1; Qualifier output uint8; DebStep input uint16; ErrAcc local single; SvcClr input

== stateflow chart SF045A_HwAgSysArbn/HwAgSysArbn/HwAgSysArbnInit1/Kinematic Integrity/SetNtcSts/ISO Fault Debounce Design ==
  note: NTCSTS_PASSD           (0)
      | NTCSTS_FAILD             (1)
      | NTCSTS_PREPASSD   (2)
      | NTCSTS_PREFAILD     (3)
      |
      | SIGQLFR_NORES        (0)
      | SIGQLFR_PASSD         (1)
      | SIGQLFR_FAILD           (2)
  note: Pass Loop
  note: Fail Loop
  note: 
  (default) -> (junction 89)
  (junction 89) -> (junction 95) [order 1] : [NtcSts ==3]
  (junction 89) -> (junction 93) [order 2] : [NtcSts ==2]
  (junction 89) -> (junction 141) [order 3] : [NtcSts ==1]
      | { ErrAcc = 32767;
      | Qualifier =2;
      |  }
  (junction 89) -> (junction 141) [order 4] : [NtcSts ==0]
      | { ErrAcc = -32768;
      | Qualifier=1;
      | }
  (junction 95) -> (junction 103) [order 2]
  (junction 95) -> (junction 111) [order 1] : [ErrAcc <=0]
      | {ErrAcc = DebStep;}
  (junction 93) -> (junction 123) [order 2] : {
      | ErrAcc = ErrAcc - DebStep;
      | }
  (junction 93) -> (junction 123) [order 1] : [(ErrAcc - DebStep) <= -32768]
      | { ErrAcc = -32768;
      | Qualifier=1;
      | }
  (junction 103) -> (junction 111) [order 1] : [(ErrAcc + DebStep) <32767]
      | {ErrAcc = ErrAcc + DebStep;}
  (junction 103) -> (junction 111) [order 2] : {ErrAcc = 32767;
      | Qualifier =2;}
  (junction 123) -> (junction 141)
  (junction 111) -> (junction 141)
  (junction 141) -> (junction 159) [order 2] : {ErrAcc = 0;
      | Qualifier =0;
      | }
  (junction 141) -> (junction 159) [order 1] : [SvcClr ==0]
  data: NtcSts input Enum: NtcSts1; Qualifier output uint8; DebStep input uint16; ErrAcc local single; SvcClr input

== stateflow chart SF045A_HwAgSysArbn/HwAgSysArbn/HwAgSysArbnPer1/HwAgArbn/VldtSnsrlsData/ThdExcdd/Kinematic Integrity/SetNtcSts/ISO Fault Debounce Design ==
  note: NTCSTS_PASSD           (0)
      | NTCSTS_FAILD             (1)
      | NTCSTS_PREPASSD   (2)
      | NTCSTS_PREFAILD     (3)
      |
      | SIGQLFR_NORES        (0)
      | SIGQLFR_PASSD         (1)
      | SIGQLFR_FAILD           (2)
  note: Pass Loop
  note: Fail Loop
  note: 
  (default) -> (junction 89)
  (junction 89) -> (junction 95) [order 1] : [NtcSts ==3]
  (junction 89) -> (junction 93) [order 2] : [NtcSts ==2]
  (junction 89) -> (junction 141) [order 3] : [NtcSts ==1]
      | { ErrAcc = 32767;
      | Qualifier =2;
      |  }
  (junction 89) -> (junction 141) [order 4] : [NtcSts ==0]
      | { ErrAcc = -32768;
      | Qualifier=1;
      | }
  (junction 95) -> (junction 103) [order 2]
  (junction 95) -> (junction 111) [order 1] : [ErrAcc <=0]
      | {ErrAcc = DebStep;}
  (junction 93) -> (junction 123) [order 2] : {
      | ErrAcc = ErrAcc - DebStep;
      | }
  (junction 93) -> (junction 123) [order 1] : [(ErrAcc - DebStep) <= -32768]
      | { ErrAcc = -32768;
      | Qualifier=1;
      | }
  (junction 103) -> (junction 111) [order 1] : [(ErrAcc + DebStep) <32767]
      | {ErrAcc = ErrAcc + DebStep;}
  (junction 103) -> (junction 111) [order 2] : {ErrAcc = 32767;
      | Qualifier =2;}
  (junction 123) -> (junction 141)
  (junction 111) -> (junction 141)
  (junction 141) -> (junction 159) [order 2] : {ErrAcc = 0;
      | Qualifier =0;
      | }
  (junction 141) -> (junction 159) [order 1] : [SvcClr ==0]
  data: NtcSts input Enum: NtcSts1; Qualifier output uint8; DebStep input uint16; ErrAcc local single; SvcClr input
